simulink model "testModel_Rx64Tx64"  (R2019a)
settings: Solver=FixedStepDiscrete  StartTime=0.0  StopTime=10.0  RelTol=1e-3
libraries: simulink x1
settings Model: DataTypeOverride=Off  Creator=tcollins  LastModifiedBy=tcollins
settings DataIOCC: LimitDataPoints=on  SaveOutput=off  SaveTime=off  ReturnWorkspaceOutputs=off
settings OptimizationCC: BlockReduction=off  ConditionallyExecuteInputs=off  DefaultParameterBehavior=Inlined  LifeSpan=inf
settings DebuggingCC: AlgebraicLoopMsg=error  SingleTaskRateTransMsg=error  AllowSymbolicDim=off  StrictBusMsg=ErrorOnBusTreatedAsVector  SFUnexpectedBacktrackingDiag=warning  SFNoUnconditionalDefaultTransitionDiag=warning  SFExecutionAtInitializationDiag=none  ArithmeticOperatorsInVariantConditions=warning
settings HardwareCC: ProdBitPerPointer=32  ProdBitPerSizeT=32  ProdBitPerPtrDiffT=32  ProdLargestAtomicFloat=None  ProdIntDivRoundTo=Undefined  ProdEndianess=Unspecified  ProdWordSize=32  ProdHWDeviceType=ASIC/FPGA->ASIC/FPGA  ProdEqTarget=off
settings SFSimCC: SimUseLocalCustomCode=off
settings RTWCC: RTWUseLocalCustomCode=off
settings CodeAppCC: StateflowObjectComments=on
settings GRTTargetCC: TargetLangStandard=C89/C90 (ANSI)  GeneratePreprocessorConditionals=Disable all
settings ConfigComp: CovScope=ReferencedModels  CovMetricSettings=dw  CovHtmlReporting=on  CovSaveCumulativeToWorkspaceVar=on  CovSaveSingleToWorkspaceVar=on  CovExternalEMLEnable=off  CovSFcnEnable=off

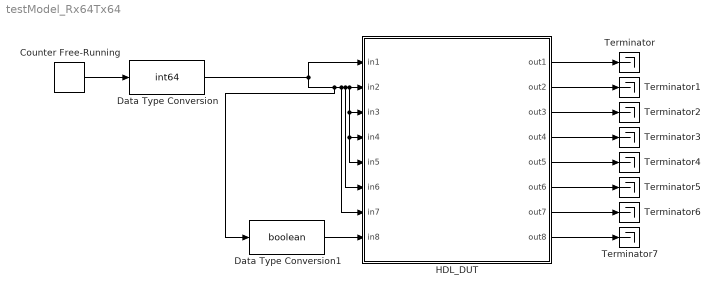
== system testModel_Rx64Tx64 ==
  Counter Free-Running : simulink/Sources/Counter Free-Running  NumBits=10  tsamp=1
  Data Type Conversion : DataTypeConversion  OutDataTypeStr=int64
  Data Type Conversion1 : DataTypeConversion  OutDataTypeStr=boolean
  HDL_DUT : Subsystem  TreatAsAtomicUnit=on
  Terminator{,1..7} (8 alike) : Terminator
  wires:
  Counter Free-Running/1 -> Data Type Conversion/1
  HDL_DUT/1(out1) -> Terminator/1
  HDL_DUT/2(out2) -> Terminator1/1
  HDL_DUT/3(out3) -> Terminator2/1
  HDL_DUT/4(out4) -> Terminator3/1
  Data Type Conversion/1 -> HDL_DUT/1(in1), HDL_DUT/2(in2), HDL_DUT/3(in3), HDL_DUT/4(in4), HDL_DUT/5(in5), HDL_DUT/6(in6), HDL_DUT/7(in7), Data Type Conversion1/1
  HDL_DUT/5(out5) -> Terminator4/1
  HDL_DUT/6(out6) -> Terminator5/1
  HDL_DUT/7(out7) -> Terminator6/1
  HDL_DUT/8(out8) -> Terminator7/1
  Data Type Conversion1/1 -> HDL_DUT/8(in8)

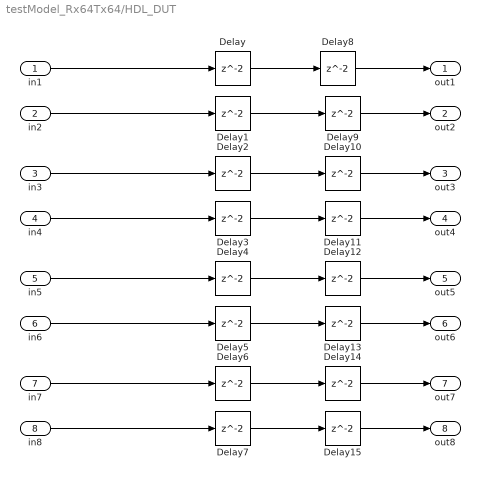
== system testModel_Rx64Tx64/HDL_DUT ==
  in1 : Inport
  in2 : Inport  Port=2
  in3 : Inport  Port=3
  in4 : Inport  Port=4
  in5 : Inport  Port=5
  in6 : Inport  Port=6
  in7 : Inport  Port=7
  in8 : Inport  Port=8
  Delay{,1..15} (16 alike) : Delay
  out1 : Outport
  out2 : Outport  Port=2
  out3 : Outport  Port=3
  out4 : Outport  Port=4
  out5 : Outport  Port=5
  out6 : Outport  Port=6
  out7 : Outport  Port=7
  out8 : Outport  Port=8
  wires:
  in1/1 -> Delay/1
  Delay/1 -> Delay8/1
  Delay1/1 -> Delay9/1
  in2/1 -> Delay1/1
  Delay3/1 -> Delay11/1
  in3/1 -> Delay2/1
  in4/1 -> Delay3/1
  Delay2/1 -> Delay10/1
  Delay6/1 -> Delay14/1
  Delay5/1 -> Delay13/1
  in7/1 -> Delay6/1
  in8/1 -> Delay7/1
  in5/1 -> Delay4/1
  in6/1 -> Delay5/1
  Delay4/1 -> Delay12/1
  Delay7/1 -> Delay15/1
  Delay8/1 -> out1/1
  Delay9/1 -> out2/1
  Delay10/1 -> out3/1
  Delay11/1 -> out4/1
  Delay12/1 -> out5/1
  Delay13/1 -> out6/1
  Delay14/1 -> out7/1
  Delay15/1 -> out8/1
